simulink model "motor_inducao"  (R2022b)
settings: Solver=ode45  StartTime=0.0  StopTime=0.3  RelTol=1e-9  EnableMultiTasking=on
values from neighbouring files (symbols this model uses):
  Bm = 0    [var_motor_1.m]    (also in var_motor_2.m = 0.0004; var_motor_3.m = 0.0001)
  f = 60    [var_motor_1.m]    (also in var_motor_2.m; var_motor_3.m)
  J = 1.662    [var_motor_1.m]    (also in var_motor_2.m = 0.002; var_motor_3.m = 0.001)
  Kabc = [1, 0; -1/2, -sqrt( 3 )/2; -1/2, sqrt( 3 )/2 ]    [var_motor_1.m]    (also in var_motor_2.m; var_motor_3.m)
  KS = [ 1, 0, 0 ; 0, -1/sqrt( 3 ), 1/sqrt( 3 ) ]    [var_motor_1.m]    (also in var_motor_2.m; var_motor_3.m)
  Lm = 34.7e-03    (= 0.0347)    [var_motor_1.m]    (also in var_motor_2.m = 0.1; var_motor_3.m = 0.37)
  Lr = Lm + Llr    (= 0.0355)    [var_motor_1.m]    (also in var_motor_2.m = 0.11; var_motor_3.m = 0.402)
  Ls = Lm + Lls    (= 0.0355)    [var_motor_1.m]    (also in var_motor_2.m = 0.11; var_motor_3.m = 0.402)
  P = 4    [var_motor_1.m]    (also in var_motor_2.m = 2; var_motor_3.m = 2)
  phi_a = 0    [var_motor_1.m]    (also in var_motor_2.m; var_motor_3.m)
  phi_b = -( 2*pi/3)    (= -2.09439510239)    [var_motor_1.m]    (also in var_motor_2.m; var_motor_3.m)
  phi_c = +( 2*pi/3 )    (= 2.09439510239)    [var_motor_1.m]    (also in var_motor_2.m; var_motor_3.m)
  Rr = 0.228    [var_motor_1.m]    (also in var_motor_2.m = 1; var_motor_3.m = 7.1)
  Rs = 0.087    [var_motor_1.m]    (also in var_motor_2.m = 0.8; var_motor_3.m = 9.4)
  TL = 100    [var_motor_1.m]    (also in var_motor_2.m = 20; var_motor_3.m = 0)
  Vm = ( 4/pi ) * 460    (= 585.690190578)    [var_motor_1.m]    (also in var_motor_2.m = 220*sqrt(2); var_motor_3.m = 220*sqrt(2))
  we = 4*pi*f / P    (= 188.495559215)    [var_motor_1.m]    (also in var_motor_2.m = 376.991118431; var_motor_3.m = 376.991118431)
settings Model: Creator=11802972  LastModifiedBy=andre
settings SolverCC: AlgebraicLoopSolver=TrustRegion
settings DataIOCC: LimitDataPoints=on  SaveFormat=Array  ReturnWorkspaceOutputs=off
settings OptimizationCC: LifeSpan=inf
settings DebuggingCC: UnconnectedInputMsg=warning  UnconnectedOutputMsg=warning  UnconnectedLineMsg=warning  SFUnexpectedBacktrackingDiag=warning  SFNoUnconditionalDefaultTransitionDiag=warning  SFExecutionAtInitializationDiag=none  SFMachineParentedDataDiag=warning  ArithmeticOperatorsInVariantConditions=warning
settings HardwareCC: ProdBitPerPointer=32  ProdBitPerSizeT=32  ProdBitPerPtrDiffT=32  ProdLargestAtomicFloat=None  ProdIntDivRoundTo=Undefined  ProdEndianess=Unspecified  ProdWordSize=32  ProdHWDeviceType=32-bit Generic
settings ModelReferenceCC: PropagateSignalLabelsOutOfModel=off
settings SFSimCC: SimUseLocalCustomCode=off  CustomCodeUndefinedFunction=UseInterfaceOnly
settings RTWCC: RTWUseLocalCustomCode=off
settings CodeAppCC: StateflowObjectComments=on
settings GRTTargetCC: TargetLangStandard=C89/C90 (ANSI)
settings ConfigComp: CovMetricSettings=dw  CovSaveCumulativeToWorkspaceVar=on  CovSaveSingleToWorkspaceVar=on  CovExternalEMLEnable=off

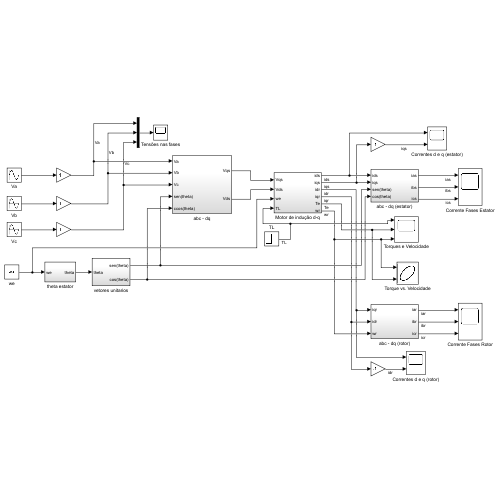
[thumbnail: Simulink's stored preview of the top-level diagram]
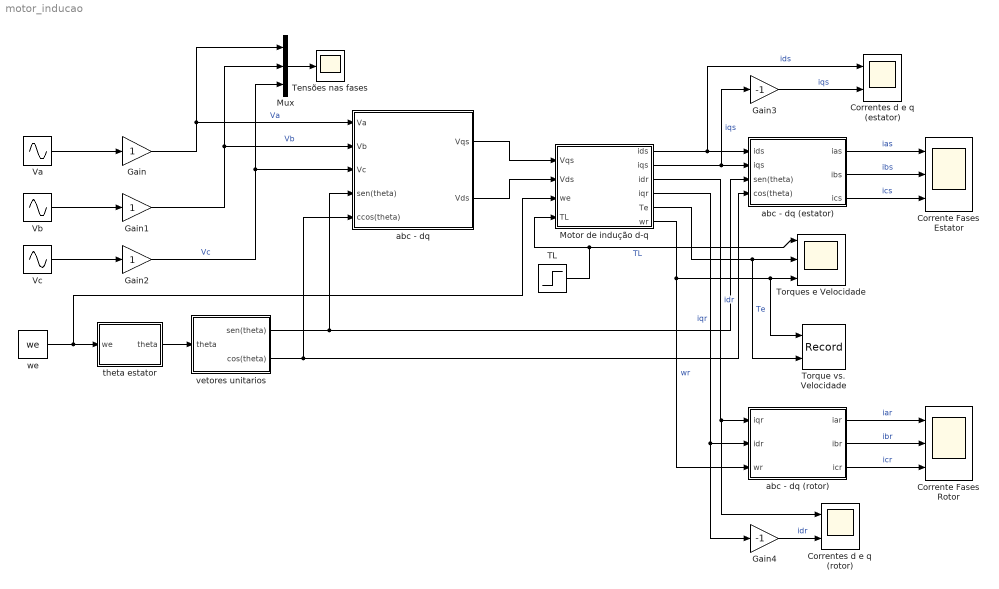
== system motor_inducao ==
  Corrente Fases Estator : Scope  NumInputPorts=3
  Corrente Fases Rotor : Scope  NumInputPorts=3
  Correntes d e q (estator) : Scope  NumInputPorts=2
  Correntes d e q (rotor) : Scope  NumInputPorts=2
  Gain : Gain
  Gain1 : Gain
  Gain2 : Gain
  Gain3 : Gain  Gain=-1
  Gain4 : Gain  Gain=-1
  Motor de indução d-q : Subsystem
  Mux : Mux  Inputs=3
  TL : Step  Time=t  After=TL  SampleTime=0
  Tensões nas fases : Scope
  Torque vs. Velocidade : Record  FileSettingsInternal="{\"entries\":[{\"content\":{\"excelSettings\":{\"content\":{},\"type\":\"Streamout.ExcelSettings\"}},\"type\":\"Streamout.FileSettingStorage\",\"uuid\":\"\"}],\"packageUris\":[\"http:\\/\\/schema.mathworks.com\\/mf0\\/streamout_blocks\\/R2020a\"],\"version\":\"1.0\"}"  Layout=[1 1]  SignalsInternal="{\"entries\":[{\"content\":{\"signals\":[{\"content\":{\"blockPath\":[],\"channel\":[],\"dimensions\":[1],\"domain\":\"\",\"lineColor\":\"#a2142f\",\"plots\":[1],\"port\":1,\"sid\":[\"\"],\"signalID\":477,\"signalName\":\"wr\"},\"type\":\"RecordBlkView.Signal\",\"uuid\":\"\"},{\"content\":{\"blockPath\":[],\"channel\":[],\"dimensions\":[1],\"domain\":\"\",\"lineColor\":\"#139fff\",\"plots\":[1],\"port\":2,\"sid\":[\"\"],\"signalID\":481,\"signalName\":\"Te\"},\"type\":\"RecordBlkView.Signal\",\"uuid\":\"\"}]},\"type\":\"RecordBlkView.InputSignals\",\"uuid\":\"\"}],\"packageUris\":[\"http:\\/\\/schema.mathworks.com\\/mf0\\/streamout_blocks\\/R2020a\"],\"version\":\"1.0\"}"  VisualizationBindings="{\"xyplotplugin\":{\"info\":[{\"series\":[{\"bindingParametersList\":[{\"parameter\":\"X-Axis\",\"signalID\":477,\"signalName\":\"wr\"},{\"parameter\":\"Y-Axis\",\"signalID\":481,\"signalName\":\"Te\"}],\"seriesID\":36260}],\"subplotID\":1}]}}"  CompatibilityTag=XY
  Torques e Velocidade : Scope  NumInputPorts=3
  Va : Sin  Amplitude=Vm  Frequency=2*pi*f  Phase=phi_a  SampleTime=0
  Vb : Sin  Amplitude=Vm  Frequency=2*pi*f  Phase=phi_b  SampleTime=0
  Vc : Sin  Amplitude=Vm  Frequency=2*pi*f  Phase=phi_c  SampleTime=0
  abc - dq : Subsystem
  abc - dq (estator) : Subsystem
  abc - dq (rotor) : Subsystem
  theta estator : Subsystem
  vetores unitarios : Subsystem
  we : Constant  Value=we
  wires:
  Va/1 -> Gain/1
  Vb/1 -> Gain1/1
  Vc/1 -> Gain2/1
  Gain/1 -> Mux/1, abc - dq/1(Va)  "Va"
  Gain1/1 -> Mux/2, abc - dq/2(Vb)  "Vb"
  Gain2/1 -> Mux/3, abc - dq/3(Vc)  "Vc"
  vetores unitarios/1(sen(theta)) -> abc - dq (estator)/3(sen(theta)), abc - dq/4(sen(theta))
  vetores unitarios/2(cos(theta)) -> abc - dq/5(ccos(theta)), abc - dq (estator)/4(cos(theta))
  theta estator/1(theta) -> vetores unitarios/1(theta)
  abc - dq/1(Vqs) -> Motor de indução d-q/1(Vqs)
  abc - dq/2(Vds) -> Motor de indução d-q/2(Vds)
  TL/1 -> Motor de indução d-q/4(TL), Torques e Velocidade/1  "TL"
  we/1 -> Motor de indução d-q/3(we), theta estator/1(we)
  Motor de indução d-q/1(ids) -> Correntes d e q (estator)/1, abc - dq (estator)/1(ids)  "ids"
  Motor de indução d-q/2(iqs) -> Gain3/1, abc - dq (estator)/2(iqs)  "iqs"
  Motor de indução d-q/3(idr) -> Correntes d e q (rotor)/1, abc - dq (rotor)/1(iqr)  "idr"
  Motor de indução d-q/4(iqr) -> Gain4/1, abc - dq (rotor)/2(idr)  "iqr"
  abc - dq (estator)/2(ibs) -> Corrente Fases Estator/2  "ibs"
  abc - dq (estator)/1(ias) -> Corrente Fases Estator/1  "ias"
  abc - dq (estator)/3(ics) -> Corrente Fases Estator/3  "ics"
  Motor de indução d-q/6(wr) -> abc - dq (rotor)/3(wr), Torque vs. Velocidade/1, Torques e Velocidade/3  "wr"
  Motor de indução d-q/5(Te) -> Torque vs. Velocidade/2, Torques e Velocidade/2  "Te"
  Mux/1 -> Tensões nas fases/1
  abc - dq (rotor)/1(iar) -> Corrente Fases Rotor/1  "iar"
  abc - dq (rotor)/2(ibr) -> Corrente Fases Rotor/2  "ibr"
  abc - dq (rotor)/3(icr) -> Corrente Fases Rotor/3  "icr"
  Gain3/1 -> Correntes d e q (estator)/2  "iqs"
  Gain4/1 -> Correntes d e q (rotor)/2  "idr"

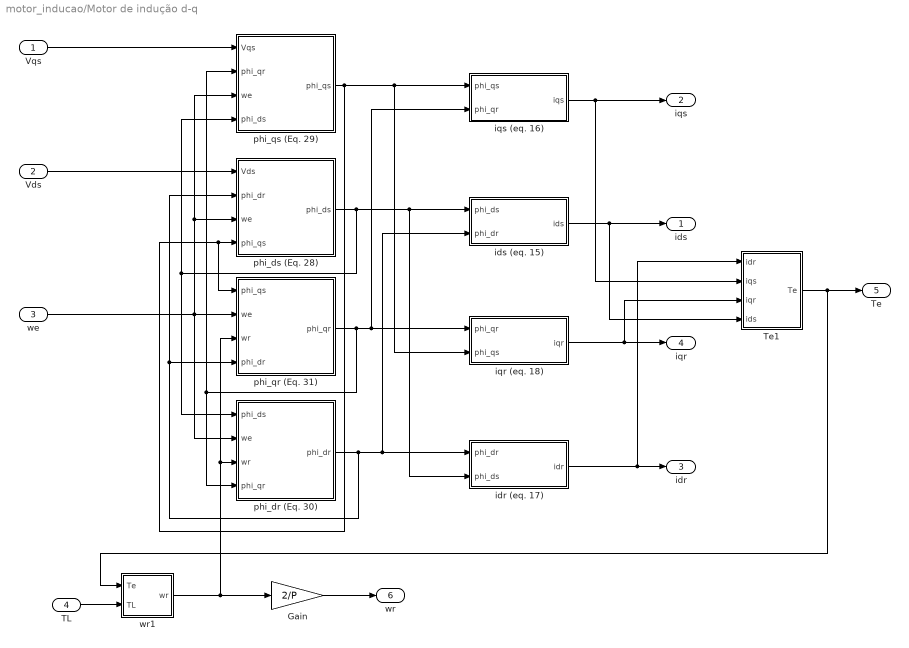
== system motor_inducao/Motor de indução d-q ==
  Vqs : Inport
  Vds : Inport  Port=2
  we : Inport  Port=3
  TL : Inport  Port=4
  Gain : Gain  Gain=2/P
  Te1 : Subsystem
  idr (eq. 17) : Subsystem
  ids (eq. 15) : Subsystem
  iqr (eq. 18) : Subsystem
  iqs (eq. 16) : Subsystem
  phi_dr (Eq. 30) : Subsystem
  phi_ds (Eq. 28) : Subsystem
  phi_qr (Eq. 31) : Subsystem
  phi_qs (Eq. 29) : Subsystem
  wr1 : Subsystem
  ids : Outport
  iqs : Outport  Port=2
  idr : Outport  Port=3
  iqr : Outport  Port=4
  Te : Outport  Port=5
  wr : Outport  Port=6
  wires:
  phi_qs (Eq. 29)/1(phi_qs) -> phi_qr (Eq. 31)/1(phi_qs), phi_ds (Eq. 28)/4(phi_qs), iqr (eq. 18)/2(phi_qs), iqs (eq. 16)/1(phi_qs)
  phi_ds (Eq. 28)/1("phi_ds ") -> phi_qs (Eq. 29)/4(phi_ds), phi_dr (Eq. 30)/1(phi_ds), idr (eq. 17)/2(phi_ds), ids (eq. 15)/1(phi_ds)
  phi_qr (Eq. 31)/1("phi_qr ") -> phi_qs (Eq. 29)/2(phi_qr), phi_dr (Eq. 30)/4(phi_qr), iqs (eq. 16)/2(phi_qr), iqr (eq. 18)/1(phi_qr)
  phi_dr (Eq. 30)/1("phi_dr ") -> ids (eq. 15)/2(phi_dr), idr (eq. 17)/1(phi_dr), phi_qr (Eq. 31)/4(phi_dr), phi_ds (Eq. 28)/2(phi_dr)
  iqs (eq. 16)/1(iqs) -> Te1/2(iqs), iqs/1
  ids (eq. 15)/1(ids) -> ids/1, Te1/4(ids)
  iqr (eq. 18)/1(iqr) -> Te1/3(iqr), iqr/1
  idr (eq. 17)/1(idr) -> idr/1, Te1/1(idr)
  Gain/1 -> wr/1
  wr1/1(wr) -> phi_qr (Eq. 31)/3(wr), phi_dr (Eq. 30)/3(wr), Gain/1
  TL/1 -> wr1/2(TL)
  Vqs/1 -> phi_qs (Eq. 29)/1(Vqs)
  Vds/1 -> phi_ds (Eq. 28)/1(Vds)
  we/1 -> phi_qr (Eq. 31)/2(we), phi_dr (Eq. 30)/2(we), phi_ds (Eq. 28)/3(we), phi_qs (Eq. 29)/3(we)
  Te1/1(Te) -> wr1/1(Te), Te/1

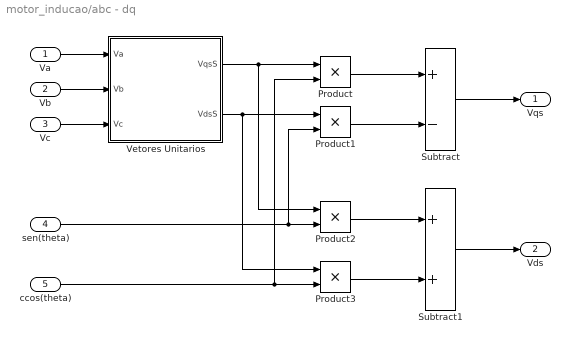
== system motor_inducao/abc - dq ==
  Va : Inport
  Vb : Inport  Port=2
  Vc : Inport  Port=3
  sen(theta) : Inport  Port=4
  ccos(theta) : Inport  Port=5
  Product{,1..3} (4 alike) : Product
  Subtract : Sum  Inputs=+-
  Subtract1 : Sum
  Vetores Unitarios : Subsystem
  Vqs : Outport
  Vds : Outport  Port=2
  wires:
  Va/1 -> Vetores Unitarios/1(Va)
  Vb/1 -> Vetores Unitarios/2(Vb)
  Vc/1 -> Vetores Unitarios/3(Vc)
  Vetores Unitarios/1(VqsS) -> Product2/1, Product/1
  Product/1 -> Subtract/1
  Subtract/1 -> Vqs/1
  Product1/1 -> Subtract/2
  Product2/1 -> Subtract1/1
  Product3/1 -> Subtract1/2
  Subtract1/1 -> Vds/1
  sen(theta)/1 -> Product1/2, Product2/2
  ccos(theta)/1 -> Product/2, Product3/2
  Vetores Unitarios/2(VdsS) -> Product3/1, Product1/1

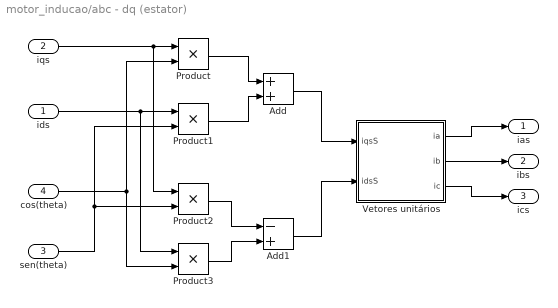
== system motor_inducao/abc - dq (estator) ==
  ids : Inport
  iqs : Inport  Port=2
  sen(theta) : Inport  Port=3
  cos(theta) : Inport  Port=4
  Add : Sum
  Add1 : Sum  Inputs=-+
  Product{,1..3} (4 alike) : Product
  Vetores unitários : Subsystem
  ias : Outport
  ibs : Outport  Port=2
  ics : Outport  Port=3
  wires:
  ids/1 -> Product3/1, Product1/1
  iqs/1 -> Product2/1, Product/1
  Product/1 -> Add/1
  Product1/1 -> Add/2
  cos(theta)/1 -> Product/2, Product3/2
  sen(theta)/1 -> Product2/2, Product1/2
  Product2/1 -> Add1/1
  Product3/1 -> Add1/2
  Vetores unitários/1(ia) -> ias/1
  Vetores unitários/2(ib) -> ibs/1
  Vetores unitários/3(ic) -> ics/1
  Add/1 -> Vetores unitários/1(iqsS)
  Add1/1 -> Vetores unitários/2(idsS)

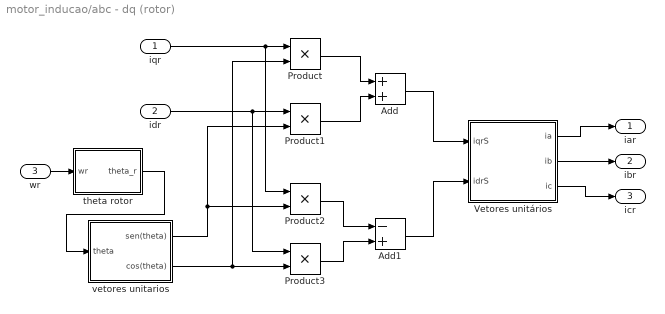
== system motor_inducao/abc - dq (rotor) ==
  iqr : Inport
  idr : Inport  Port=2
  wr : Inport  Port=3
  Add : Sum
  Add1 : Sum  Inputs=-+
  Product{,1..3} (4 alike) : Product
  Vetores unitários : Subsystem
  theta rotor : Subsystem
  vetores unitarios : Subsystem
  iar : Outport
  ibr : Outport  Port=2
  icr : Outport  Port=3
  wires:
  wr/1 -> theta rotor/1(wr)
  Add1/1 -> Vetores unitários/2(idrS)
  Product1/1 -> Add/2
  Product2/1 -> Add1/1
  idr/1 -> Product3/1, Product1/1
  Product/1 -> Add/1
  Add/1 -> Vetores unitários/1(iqrS)
  iqr/1 -> Product2/1, Product/1
  Product3/1 -> Add1/2
  theta rotor/1(theta_r) -> vetores unitarios/1(theta)
  Vetores unitários/1(ia) -> iar/1
  Vetores unitários/2(ib) -> ibr/1
  Vetores unitários/3(ic) -> icr/1
  vetores unitarios/1(sen(theta)) -> Product2/2, Product1/2
  vetores unitarios/2(cos(theta)) -> Product/2, Product3/2

== system motor_inducao/theta estator ==
  we : Inport
  Integrator : Integrator
  theta : Outport
  wires:
  we/1 -> Integrator/1
  Integrator/1 -> theta/1

== system motor_inducao/vetores unitarios ==
  theta : Inport
  Trigonometric Function : Trigonometry
  Trigonometric Function1 : Trigonometry  Operator=cos
  sen(theta) : Outport
  cos(theta) : Outport  Port=2
  wires:
  Trigonometric Function/1 -> sen(theta)/1
  Trigonometric Function1/1 -> cos(theta)/1
  theta/1 -> Trigonometric Function/1, Trigonometric Function1/1

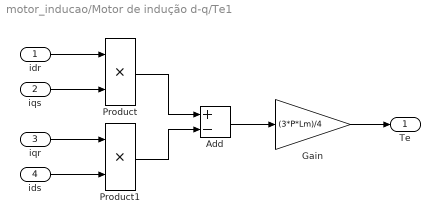
== system motor_inducao/Motor de indução d-q/Te1 ==
  idr : Inport
  iqs : Inport  Port=2
  iqr : Inport  Port=3
  ids : Inport  Port=4
  Add : Sum  Inputs=+-
  Gain : Gain  Gain=(3*P*Lm)/4
  Product : Product
  Product1 : Product
  Te : Outport
  wires:
  idr/1 -> Product/1
  iqs/1 -> Product/2
  iqr/1 -> Product1/1
  ids/1 -> Product1/2
  Product/1 -> Add/1
  Product1/1 -> Add/2
  Add/1 -> Gain/1
  Gain/1 -> Te/1

== system motor_inducao/Motor de indução d-q/idr (eq. 17) ==
  phi_dr : Inport
  phi_ds : Inport  Port=2
  Gain : Gain  Gain=Ls/((Lr*Ls)-Lm^2)
  Gain1 : Gain  Gain=Lm/((Lr*Ls)-Lm^2)
  Subtract : Sum  Inputs=+-
  idr : Outport
  wires:
  phi_dr/1 -> Gain/1
  phi_ds/1 -> Gain1/1
  Gain/1 -> Subtract/1
  Gain1/1 -> Subtract/2
  Subtract/1 -> idr/1

== system motor_inducao/Motor de indução d-q/ids (eq. 15) ==
  phi_ds : Inport
  phi_dr : Inport  Port=2
  Gain : Gain  Gain=Lr/((Lr*Ls)-Lm^2)
  Gain1 : Gain  Gain=Lm/((Lr*Ls)-Lm^2)
  Subtract : Sum  Inputs=+-
  ids : Outport
  wires:
  phi_ds/1 -> Gain/1
  phi_dr/1 -> Gain1/1
  Gain/1 -> Subtract/1
  Gain1/1 -> Subtract/2
  Subtract/1 -> ids/1

== system motor_inducao/Motor de indução d-q/iqr (eq. 18) ==
  phi_qr : Inport
  phi_qs : Inport  Port=2
  Gain : Gain  Gain=Ls/((Lr*Ls)-Lm^2)
  Gain1 : Gain  Gain=Lm/((Lr*Ls)-Lm^2)
  Subtract : Sum  Inputs=+-
  iqr : Outport
  wires:
  phi_qr/1 -> Gain/1
  phi_qs/1 -> Gain1/1
  Gain/1 -> Subtract/1
  Gain1/1 -> Subtract/2
  Subtract/1 -> iqr/1

== system motor_inducao/Motor de indução d-q/iqs (eq. 16) ==
  phi_qs : Inport
  phi_qr : Inport  Port=2
  Gain : Gain  Gain=Lr/((Lr*Ls)-Lm^2)
  Gain1 : Gain  Gain=Lm/((Lr*Ls)-Lm^2)
  Subtract : Sum  Inputs=+-
  iqs : Outport
  wires:
  phi_qs/1 -> Gain/1
  phi_qr/1 -> Gain1/1
  Gain/1 -> Subtract/1
  Gain1/1 -> Subtract/2
  Subtract/1 -> iqs/1

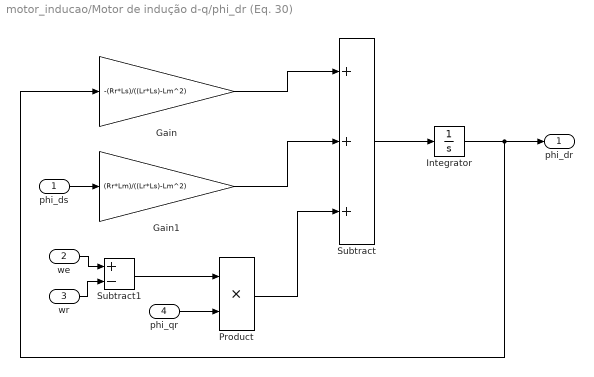
== system motor_inducao/Motor de indução d-q/phi_dr (Eq. 30) ==
  phi_ds : Inport
  we : Inport  Port=2
  wr : Inport  Port=3
  phi_qr : Inport  Port=4
  Gain : Gain  Gain=-(Rr*Ls)/((Lr*Ls)-Lm^2)
  Gain1 : Gain  Gain=(Rr*Lm)/((Lr*Ls)-Lm^2)
  Integrator : Integrator
  Product : Product
  Subtract : Sum  Inputs=+++
  Subtract1 : Sum  Inputs=+-
  "phi_dr " : Outport
  wires:
  Subtract/1 -> Integrator/1
  Integrator/1 -> "phi_dr "/1, Gain/1
  phi_ds/1 -> Gain1/1
  Subtract1/1 -> Product/1
  phi_qr/1 -> Product/2
  Gain/1 -> Subtract/1
  Gain1/1 -> Subtract/2
  Product/1 -> Subtract/3
  we/1 -> Subtract1/1
  wr/1 -> Subtract1/2

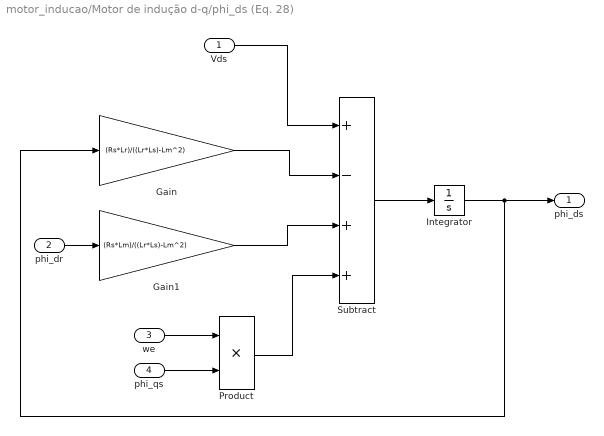
== system motor_inducao/Motor de indução d-q/phi_ds (Eq. 28) ==
  Vds : Inport
  phi_dr : Inport  Port=2
  we : Inport  Port=3
  phi_qs : Inport  Port=4
  Gain : Gain  Gain=(Rs*Lr)/((Lr*Ls)-Lm^2)
  Gain1 : Gain  Gain=(Rs*Lm)/((Lr*Ls)-Lm^2)
  Integrator : Integrator
  Product : Product
  Subtract : Sum  Inputs=+-++
  "phi_ds " : Outport
  wires:
  Subtract/1 -> Integrator/1
  Integrator/1 -> "phi_ds "/1, Gain/1
  Vds/1 -> Subtract/1
  Gain/1 -> Subtract/2
  Gain1/1 -> Subtract/3
  phi_dr/1 -> Gain1/1
  we/1 -> Product/1
  phi_qs/1 -> Product/2
  Product/1 -> Subtract/4

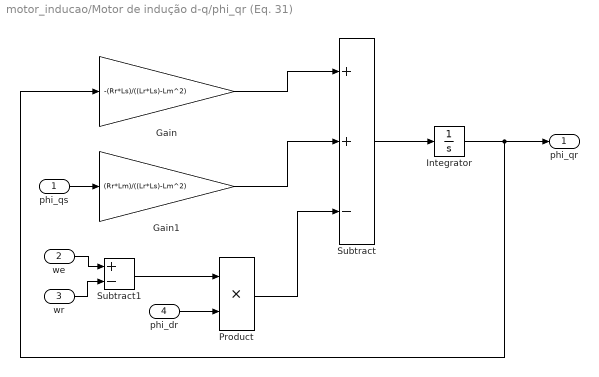
== system motor_inducao/Motor de indução d-q/phi_qr (Eq. 31) ==
  phi_qs : Inport
  we : Inport  Port=2
  wr : Inport  Port=3
  phi_dr : Inport  Port=4
  Gain : Gain  Gain=-(Rr*Ls)/((Lr*Ls)-Lm^2)
  Gain1 : Gain  Gain=(Rr*Lm)/((Lr*Ls)-Lm^2)
  Integrator : Integrator
  Product : Product
  Subtract : Sum  Inputs=++-
  Subtract1 : Sum  Inputs=+-
  "phi_qr " : Outport
  wires:
  Subtract/1 -> Integrator/1
  Integrator/1 -> "phi_qr "/1, Gain/1
  phi_qs/1 -> Gain1/1
  Subtract1/1 -> Product/1
  phi_dr/1 -> Product/2
  Gain/1 -> Subtract/1
  Gain1/1 -> Subtract/2
  Product/1 -> Subtract/3
  we/1 -> Subtract1/1
  wr/1 -> Subtract1/2

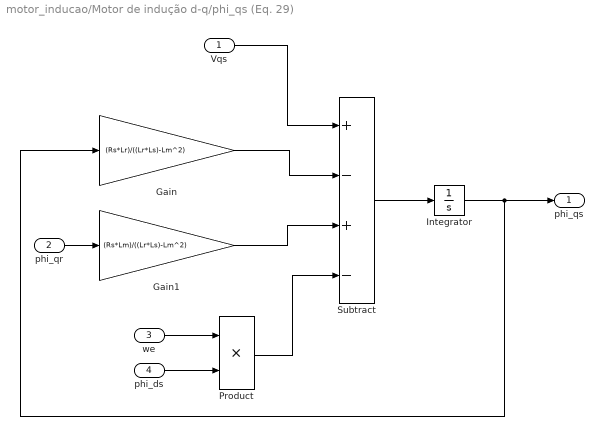
== system motor_inducao/Motor de indução d-q/phi_qs (Eq. 29) ==
  Vqs : Inport
  phi_qr : Inport  Port=2
  we : Inport  Port=3
  phi_ds : Inport  Port=4
  Gain : Gain  Gain=(Rs*Lr)/((Lr*Ls)-Lm^2)
  Gain1 : Gain  Gain=(Rs*Lm)/((Lr*Ls)-Lm^2)
  Integrator : Integrator
  Product : Product
  Subtract : Sum  Inputs=+-+-
  phi_qs : Outport
  wires:
  Subtract/1 -> Integrator/1
  Integrator/1 -> Gain/1, phi_qs/1
  Vqs/1 -> Subtract/1
  Gain/1 -> Subtract/2
  Gain1/1 -> Subtract/3
  phi_qr/1 -> Gain1/1
  we/1 -> Product/1
  phi_ds/1 -> Product/2
  Product/1 -> Subtract/4

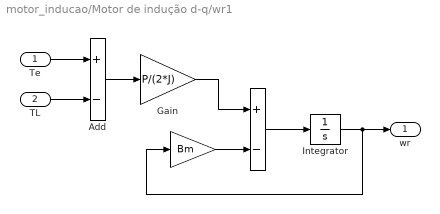
== system motor_inducao/Motor de indução d-q/wr1 ==
  Te : Inport
  TL : Inport  Port=2
  " " : Sum  Inputs=+-
  "  " : Gain  Gain=Bm
  Add : Sum  Inputs=+-
  Gain : Gain  Gain=P/(2*J)
  Integrator : Integrator
  wr : Outport
  wires:
  Te/1 -> Add/1
  TL/1 -> Add/2
  Add/1 -> Gain/1
  Integrator/1 -> "  "/1, wr/1
  " "/1 -> Integrator/1
  Gain/1 -> " "/1
  "  "/1 -> " "/2

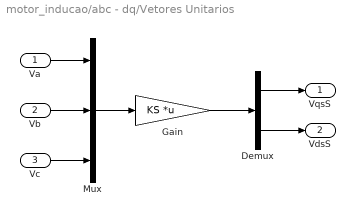
== system motor_inducao/abc - dq/Vetores Unitarios ==
  Va : Inport
  Vb : Inport  Port=2
  Vc : Inport  Port=3
  Demux : Demux  Outputs=2
  Gain : Gain  Gain=KS  Multiplication=Matrix(K*u)
  Mux : Mux  Inputs=3
  VqsS : Outport
  VdsS : Outport  Port=2
  wires:
  Va/1 -> Mux/1
  Vb/1 -> Mux/2
  Vc/1 -> Mux/3
  Mux/1 -> Gain/1
  Gain/1 -> Demux/1
  Demux/1 -> VqsS/1
  Demux/2 -> VdsS/1

== system motor_inducao/abc - dq (estator)/Vetores unitários ==
  iqsS : Inport
  idsS : Inport  Port=2
  Demux : Demux  Outputs=3
  Gain : Gain  Gain=Kabc  Multiplication=Matrix(K*u)
  Mux : Mux  Inputs=2
  ia : Outport
  ib : Outport  Port=2
  ic : Outport  Port=3
  wires:
  iqsS/1 -> Mux/1
  idsS/1 -> Mux/2
  Mux/1 -> Gain/1
  Gain/1 -> Demux/1
  Demux/1 -> ia/1
  Demux/2 -> ib/1
  Demux/3 -> ic/1

== system motor_inducao/abc - dq (rotor)/Vetores unitários ==
  iqrS : Inport
  idrS : Inport  Port=2
  Demux : Demux  Outputs=3
  Gain : Gain  Gain=Kabc  Multiplication=Matrix(K*u)
  Mux : Mux  Inputs=2
  ia : Outport
  ib : Outport  Port=2
  ic : Outport  Port=3
  wires:
  iqrS/1 -> Mux/1
  idrS/1 -> Mux/2
  Mux/1 -> Gain/1
  Gain/1 -> Demux/1
  Demux/1 -> ia/1
  Demux/2 -> ib/1
  Demux/3 -> ic/1

== system motor_inducao/abc - dq (rotor)/theta rotor ==
  wr : Inport
  Integrator : Integrator
  theta_r : Outport
  wires:
  wr/1 -> Integrator/1
  Integrator/1 -> theta_r/1

== system motor_inducao/abc - dq (rotor)/vetores unitarios ==
  theta : Inport
  Trigonometric Function : Trigonometry
  Trigonometric Function1 : Trigonometry  Operator=cos
  sen(theta) : Outport
  cos(theta) : Outport  Port=2
  wires:
  Trigonometric Function/1 -> sen(theta)/1
  Trigonometric Function1/1 -> cos(theta)/1
  theta/1 -> Trigonometric Function/1, Trigonometric Function1/1
